simulink model "mic_input_2source"  (R2013b)
settings: Solver=FixedStepDiscrete  StartTime=0.0  StopTime=.01  FixedStep=1/44100  RelTol=1e-3
libraries: dspsrcs4 x30
settings Model: Creator=nryan1_guest  LastModifiedBy=nryan1_guest

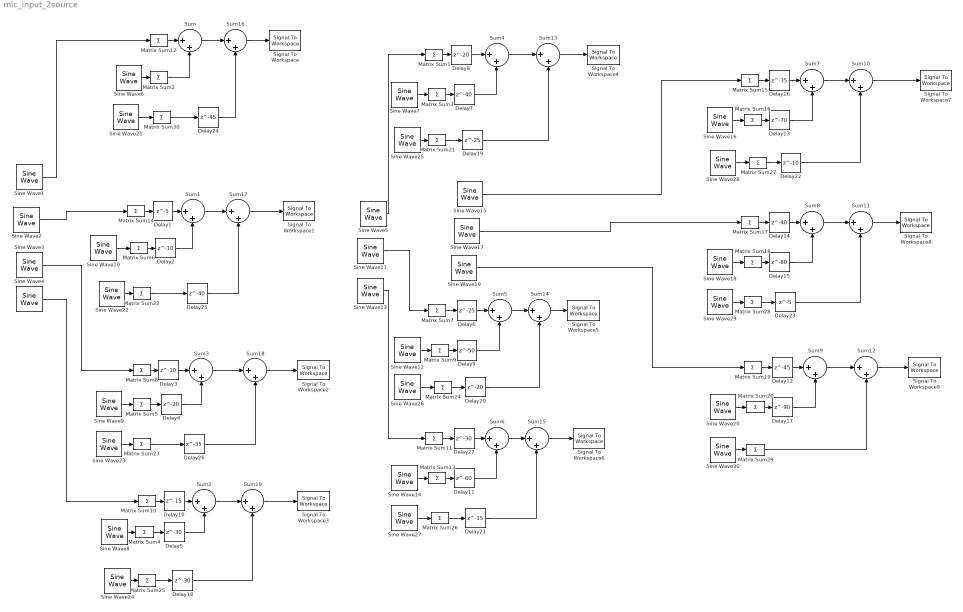
== system mic_input_2source ==
  Delay1 : Delay  DelayLength=5  InitialCondition=0
  Delay10 : Delay  DelayLength=15  InitialCondition=0
  Delay11 : Delay  DelayLength=60  InitialCondition=0
  Delay12 : Delay  DelayLength=45  InitialCondition=0
  Delay13 : Delay  DelayLength=70  InitialCondition=0
  Delay14 : Delay  DelayLength=40  InitialCondition=0
  Delay15 : Delay  DelayLength=80  InitialCondition=0
  Delay16 : Delay  DelayLength=35  InitialCondition=0
  Delay17 : Delay  DelayLength=90  InitialCondition=0
  Delay18 : Delay  DelayLength=30  InitialCondition=0
  Delay19 : Delay  DelayLength=25  InitialCondition=0
  Delay2 : Delay  DelayLength=10  InitialCondition=0
  Delay20 : Delay  DelayLength=20  InitialCondition=0
  Delay21 : Delay  DelayLength=15  InitialCondition=0
  Delay22 : Delay  DelayLength=10  InitialCondition=0
  Delay23 : Delay  DelayLength=5  InitialCondition=0
  Delay24 : Delay  DelayLength=45  InitialCondition=0
  Delay25 : Delay  DelayLength=40  InitialCondition=0
  Delay26 : Delay  DelayLength=35  InitialCondition=0
  Delay27 : Delay  DelayLength=30  InitialCondition=0
  Delay3 : Delay  DelayLength=10  InitialCondition=0
  Delay4 : Delay  DelayLength=20  InitialCondition=0
  Delay5 : Delay  DelayLength=30  InitialCondition=0
  Delay6 : Delay  DelayLength=25  InitialCondition=0
  Delay7 : Delay  DelayLength=40  InitialCondition=0
  Delay8 : Delay  DelayLength=20  InitialCondition=0
  Delay9 : Delay  DelayLength=50  InitialCondition=0
  Matrix Sum{1..30} (30 alike) : Sum  Inputs=+  CollapseMode=Specified dimension  CollapseDim=2  SampleTime=1/44100
  Signal To Workspace : SignalToWorkspace  VariableName=mic1
      settings: CopyFcn=dspblkcopystw(gcbh);
  Signal To Workspace1 : SignalToWorkspace  VariableName=mic2
      settings: CopyFcn=dspblkcopystw(gcbh);
  Signal To Workspace2 : SignalToWorkspace  VariableName=mic3
      settings: CopyFcn=dspblkcopystw(gcbh);
  Signal To Workspace3 : SignalToWorkspace  VariableName=mic4
      settings: CopyFcn=dspblkcopystw(gcbh);
  Signal To Workspace4 : SignalToWorkspace  VariableName=mic5
      settings: CopyFcn=dspblkcopystw(gcbh);
  Signal To Workspace5 : SignalToWorkspace  VariableName=mic6
      settings: CopyFcn=dspblkcopystw(gcbh);
  Signal To Workspace6 : SignalToWorkspace  VariableName=mic7
      settings: CopyFcn=dspblkcopystw(gcbh);
  Signal To Workspace7 : SignalToWorkspace  VariableName=mic8
      settings: CopyFcn=dspblkcopystw(gcbh);
  Signal To Workspace8 : SignalToWorkspace  VariableName=mic9
      settings: CopyFcn=dspblkcopystw(gcbh);
  Signal To Workspace9 : SignalToWorkspace  VariableName=mic10
      settings: CopyFcn=dspblkcopystw(gcbh);
  Sine Wave{1..5,11,13,15,17,19} (10 alike) : dspsrcs4/Sine Wave  Amplitude=5  Frequency=350  Phase=0  SampleMode=Discrete  OutComplex=Real  CompMethod=Trigonometric fcn  TableSize=Speed  SampleTime=1/44100  SamplesPerFrame=1  ResetState=Restart at time zero  dataType=double  wordLen=16  udDataType=sfix(16)  fracBitsMode=Best precision  numFracBits=15  OutDataTypeStr=double  LastOutDataTypeStr=double
  Sine Wave{6..10,12,14,16,18,20} (10 alike) : dspsrcs4/Sine Wave  Amplitude=4  Frequency=1000  Phase=0  SampleMode=Discrete  OutComplex=Real  CompMethod=Trigonometric fcn  TableSize=Speed  SampleTime=1/44100  SamplesPerFrame=1  ResetState=Restart at time zero  dataType=double  wordLen=16  udDataType=sfix(16)  fracBitsMode=Best precision  numFracBits=15  OutDataTypeStr=double  LastOutDataTypeStr=double
  Sine Wave{21..30} (10 alike) : dspsrcs4/Sine Wave  Amplitude=6  Frequency=1000  Phase=0  SampleMode=Discrete  OutComplex=Real  CompMethod=Trigonometric fcn  TableSize=Speed  SampleTime=1/44100  SamplesPerFrame=1  ResetState=Restart at time zero  dataType=double  wordLen=16  udDataType=sfix(16)  fracBitsMode=Best precision  numFracBits=15  OutDataTypeStr=double  LastOutDataTypeStr=double
  Sum{,1..19} (20 alike) : Sum  Inputs=|++
  wires:
  Sine Wave1/1 -> Matrix Sum12/1
  Sine Wave3/1 -> Matrix Sum8/1
  Sine Wave2/1 -> Matrix Sum14/1
  Sine Wave4/1 -> Matrix Sum10/1
  Sine Wave5/1 -> Matrix Sum1/1
  Sine Wave7/1 -> Matrix Sum3/1
  Sine Wave8/1 -> Matrix Sum4/1
  Sine Wave6/1 -> Matrix Sum2/1
  Sine Wave10/1 -> Matrix Sum6/1
  Sine Wave9/1 -> Matrix Sum5/1
  Matrix Sum12/1 -> Sum/1
  Matrix Sum2/1 -> Sum/2
  Matrix Sum6/1 -> Delay2/1
  Delay2/1 -> Sum1/2
  Matrix Sum5/1 -> Delay4/1
  Delay4/1 -> Sum3/2
  Matrix Sum4/1 -> Delay5/1
  Delay5/1 -> Sum2/2
  Matrix Sum3/1 -> Delay7/1
  Delay7/1 -> Sum4/2
  Sine Wave11/1 -> Matrix Sum7/1
  Sine Wave12/1 -> Matrix Sum9/1
  Matrix Sum9/1 -> Delay9/1
  Delay9/1 -> Sum5/2
  Sine Wave13/1 -> Matrix Sum11/1
  Sine Wave14/1 -> Matrix Sum13/1
  Matrix Sum13/1 -> Delay11/1
  Delay11/1 -> Sum6/2
  Sine Wave15/1 -> Matrix Sum15/1
  Sine Wave16/1 -> Matrix Sum16/1
  Matrix Sum16/1 -> Delay13/1
  Delay13/1 -> Sum7/2
  Sine Wave17/1 -> Matrix Sum17/1
  Sine Wave18/1 -> Matrix Sum18/1
  Matrix Sum18/1 -> Delay15/1
  Delay15/1 -> Sum8/2
  Sine Wave19/1 -> Matrix Sum19/1
  Sine Wave20/1 -> Matrix Sum20/1
  Matrix Sum20/1 -> Delay17/1
  Delay17/1 -> Sum9/2
  Sine Wave23/1 -> Matrix Sum23/1
  Sine Wave24/1 -> Matrix Sum25/1
  Sine Wave27/1 -> Matrix Sum26/1
  Sine Wave26/1 -> Matrix Sum24/1
  Sine Wave25/1 -> Matrix Sum21/1
  Sine Wave21/1 -> Matrix Sum30/1
  Sine Wave22/1 -> Matrix Sum22/1
  Sine Wave28/1 -> Matrix Sum27/1
  Sine Wave29/1 -> Matrix Sum28/1
  Sine Wave30/1 -> Matrix Sum29/1
  Matrix Sum29/1 -> Sum12/2
  Sum9/1 -> Sum12/1
  Sum12/1 -> Signal To Workspace9/1
  Matrix Sum28/1 -> Delay23/1
  Delay23/1 -> Sum11/2
  Sum8/1 -> Sum11/1
  Sum11/1 -> Signal To Workspace8/1
  Matrix Sum27/1 -> Delay22/1
  Delay22/1 -> Sum10/2
  Sum7/1 -> Sum10/1
  Sum10/1 -> Signal To Workspace7/1
  Matrix Sum26/1 -> Delay21/1
  Delay21/1 -> Sum15/2
  Sum6/1 -> Sum15/1
  Sum15/1 -> Signal To Workspace6/1
  Matrix Sum24/1 -> Delay20/1
  Delay20/1 -> Sum14/2
  Sum5/1 -> Sum14/1
  Sum14/1 -> Signal To Workspace5/1
  Matrix Sum21/1 -> Delay19/1
  Sum4/1 -> Sum13/1
  Delay19/1 -> Sum13/2
  Sum13/1 -> Signal To Workspace4/1
  Matrix Sum25/1 -> Delay18/1
  Delay18/1 -> Sum19/2
  Sum2/1 -> Sum19/1
  Sum19/1 -> Signal To Workspace3/1
  Matrix Sum23/1 -> Delay26/1
  Sum3/1 -> Sum18/1
  Sum18/1 -> Signal To Workspace2/1
  Delay26/1 -> Sum18/2
  Sum1/1 -> Sum17/1
  Sum17/1 -> Signal To Workspace1/1
  Matrix Sum30/1 -> Delay24/1
  Sum/1 -> Sum16/1
  Delay24/1 -> Sum16/2
  Sum16/1 -> Signal To Workspace/1
  Matrix Sum22/1 -> Delay25/1
  Delay25/1 -> Sum17/2
  Matrix Sum14/1 -> Delay1/1
  Delay1/1 -> Sum1/1
  Matrix Sum8/1 -> Delay3/1
  Delay3/1 -> Sum3/1
  Matrix Sum10/1 -> Delay10/1
  Delay10/1 -> Sum2/1
  Matrix Sum1/1 -> Delay8/1
  Delay8/1 -> Sum4/1
  Matrix Sum7/1 -> Delay6/1
  Delay6/1 -> Sum5/1
  Matrix Sum11/1 -> Delay27/1
  Delay27/1 -> Sum6/1
  Matrix Sum15/1 -> Delay16/1
  Delay16/1 -> Sum7/1
  Matrix Sum17/1 -> Delay14/1
  Delay14/1 -> Sum8/1
  Matrix Sum19/1 -> Delay12/1
  Delay12/1 -> Sum9/1
